simulink library "vehicleWeight_cl"  (R2022a)
settings: Solver=VariableStepAuto  StartTime=0.0  StopTime=10.0  RelTol=1e-3
undefined symbols (not defined in the file): env, VEHICLE, vhcl
libraries: vrlib x2, eulAng2RotMat_ul x1, eulDot x1, tethersMoment_cl x1, thrAttachPtKinematics_ul x1
settings Model: Creator=mcobb  LastModifiedBy=lhill8
settings SolverCC: AlgebraicLoopSolver=TrustRegion
settings DebuggingCC: UnconnectedInputMsg=warning  UnconnectedOutputMsg=warning  UnconnectedLineMsg=warning  SFMachineParentedDataDiag=warning  ArithmeticOperatorsInVariantConditions=warning
settings SFSimCC: CustomCodeUndefinedFunction=UseInterfaceOnly

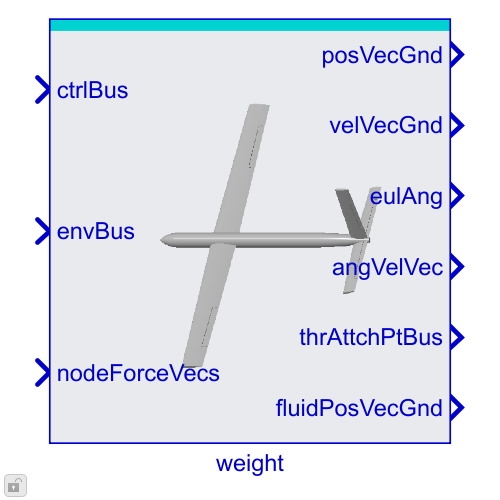
[thumbnail: Simulink's stored preview of the top-level diagram]
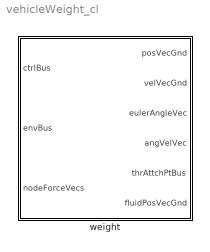
== system vehicleWeight_cl ==
  weight : Subsystem  VariantControl=strcmpi(VEHICLE,'vehicleManta2Rot')  mask{vcl=vhcl, rho=env.water.density.Value, grav=env.gravAccel.Value}
      mask prompts: vcl "Vehicle"; rho "Density"; grav "Gravity"
      mask DialogControl Container9 Prompt: General
      mask DialogControl Container5 Prompt: Vehicle object (OCT.vehicle)
      mask DialogControl ParameterGroupVar Prompt: Environment Object (OCT.env)
      mask Display:
      | image('kite2.PNG',[0 0 700 700]/4,'on')
      | 
      | port_label('input',1,'ctrlBus')
      | port_label('input',2,'envBus')
      | port_label('input',3,'nodeForceVecs')
      | 
      | port_label('output',1,'posVecGnd')
      | port_label('output',2,'velVecGnd')
      | port_label('output',3,'eulAng')
      | port_label('output',4,'angVelVec')
      | port_label('output',5,'thrAttchPtBus')
      | port_label('output',6,'fluidPosVecGnd')

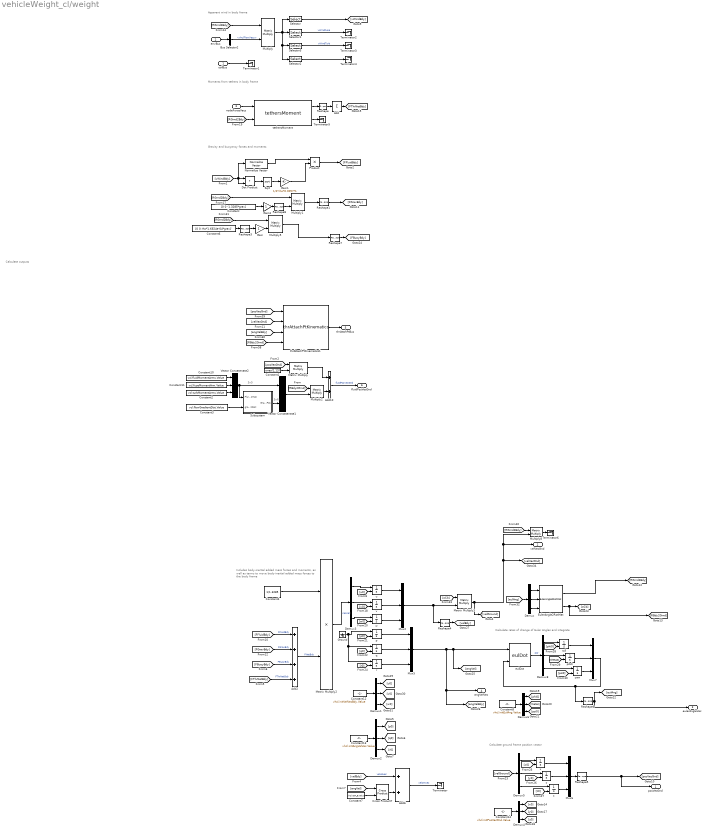
== system vehicleWeight_cl/weight ==
  note: 3x6
  note: 3x5
  note: Calculate outputs
  note: Apparent wind in body frame
  note: Gravity and buoyancy forces and moments
  note: Moments from tethers in body frame
  note: Calculate rates of change of Euler Angles and integrate
  note: Includes body-inertial added mass forces and moments,
      | as well as terms to move body-inertial added mass
      | forces to the body frame
  note: Calculate ground frame position vector
  ctrlBus : Inport
  envBus : Inport  Port=2  OutDataTypeStr=Bus: envBus
  nodeForceVecs : Inport  Port=3
  Add : Sum  Inputs=+  CollapseMode=Specified dimension  CollapseDim=2
  Add10 : Sum
  Add2 : Sum  Inputs=++++
  Add6 : Sum
  Bus Selector2 : BusSelector  OutputSignals=vhclFlowVecs
  Constant : Constant  Value=[0 0 -1.3285*grav]
  Constant1 : Constant  Value=ones(1,13)  VectorParams1D=off
  Constant10 : Constant  Value=vcl.fluidMomentArms.Value
  Constant11 : Constant  Value=vcl.fuseMomentArm.Value
  Constant12 : Constant  Value=vhcl.initVelVecBdy.Value
  Constant13 : Constant  Value=vhcl.initAngVelVec.Value
  Constant14 : Constant  Value=vhcl.initPosVecGnd.Value
  Constant2 : Constant  Value=vcl.turbMomentArms.Value
  Constant3 : Constant  Value=vcl.flowGradientDist.Value
  Constant4 : Constant  Value=1/1.3285  VectorParams1D=off
  Constant6 : Constant  Value=[0 0 rho*1.6924e-04*grav]'
  Constant7 : Constant  Value=vhcl.rCM_B.Value
  Constant8 : Constant  Value=vhcl.initEulAng.Value
  Cross Product7 : vrlib/Utilities/Cross Product
  Demux{,1..6,8} (8 alike) : Demux  Outputs=3
  Dot Product : DotProduct  OutDataTypeStr=Inherit: Inherit via internal rule
  EulerAngle2RotMat : eulAng2RotMat_ul/EulerAngle2RotMat  SystemSampleTime=-1  VariantActivationTime=update diagram  Latency=0  AutoFrameSizeCalculation=off
  Gain : Gain
  Gain1 : Gain  Gain=1/2*rho*0.0057*1
  Gain3 : Gain
  Ground : Ground
  Matrix Multiply : Product  Multiplication=Matrix(*)
  Matrix Multiply2 : Product
  Matrix Multiply3 : Product  Multiplication=Matrix(*)
  Multiply{,1..2,5,8} (5 alike) : Product  Multiplication=Matrix(*)
  Mux{2,5..7} (4 alike) : Mux  Inputs=3
  Normalize Vector : vrlib/Utilities/Normalize Vector  maxzero=0
  Product : Product
  Reshape : Reshape  OutputDimensionality=Customize  OutputDimensions=[3 vcl.numTethers.Value]
  Reshape{1,3..8} (7 alike) : Reshape  OutputDimensionality=Column vector (2-D)
  Selector : Selector  NumberOfDimensions=2  InputPortWidth=3  IndexOptions=Select all,Index vector (dialog)  Indices=[1 3],1  OutputSizes=1,1
  Selector1 : Selector  NumberOfDimensions=2  InputPortWidth=3  IndexOptions=Select all,Index vector (dialog)  Indices=[1 3],5  OutputSizes=1,1
  Selector2 : Selector  NumberOfDimensions=2  InputPortWidth=3  IndexOptions=Select all,Index vector (dialog)  Indices=[1 3],8:13  OutputSizes=1,1
  Selector3 : Selector  NumberOfDimensions=2  InputPortWidth=3  IndexOptions=Select all,Index vector (dialog)  Indices=[1 3],6:7  OutputSizes=1,1
  Sqrt : Sqrt
  Subsystem : Subsystem
  Terminator{,1..6} (7 alike) : Terminator
  Vector Concatenate1 : Concatenate  Mode=Multidimensional array  ConcatenateDimension=2
  Vector Concatenate2 : Concatenate  NumInputs=3  Mode=Multidimensional array  ConcatenateDimension=2
  eulDot : eulDot/eulDot  SystemSampleTime=-1  VariantActivationTime=update diagram  Latency=0  AutoFrameSizeCalculation=off
  p : Integrator  InitialConditionSource=external
  pitch : Integrator  InitialConditionSource=external
  q : Integrator  InitialConditionSource=external
  r : Integrator  InitialConditionSource=external
  roll : Integrator  InitialConditionSource=external
  tethersMoment : tethersMoment_cl/tethersMoment  arms=vcl.struct('OCT.thrAttch')
  thrAttachPtKinematics1 : thrAttachPtKinematics_ul/thrAttachPtKinematics  atchPts=vcl.struct('OCT.thrAttch')
  u : Integrator  InitialConditionSource=external
  v : Integrator  InitialConditionSource=external
  w : Integrator  InitialConditionSource=external
  x : Integrator  InitialConditionSource=external
  y : Integrator  InitialConditionSource=external
  yaw : Integrator  InitialConditionSource=external
  z : Integrator  InitialConditionSource=external
  posVecGnd : Outport  VectorParamsAs1DForOutWhenUnconnected=off
  velVecGnd : Outport  Port=2  VectorParamsAs1DForOutWhenUnconnected=off
  eulerAngleVec : Outport  Port=3  VectorParamsAs1DForOutWhenUnconnected=off
  angVelVec : Outport  Port=4  VectorParamsAs1DForOutWhenUnconnected=off
  thrAttchPtBus : Outport  Port=5  VectorParamsAs1DForOutWhenUnconnected=off
  fluidPosVecGnd : Outport  Port=6  VectorParamsAs1DForOutWhenUnconnected=off
  wires:
  thrAttachPtKinematics1/1 -> thrAttchPtBus/1
  Constant6/1 -> Reshape3/1
  Reshape3/1 -> Gain/1
  [RGrnd2Bdy] -> Multiply5/1
  Gain/1 -> Multiply5/2
  Multiply5/1 -> Reshape7/1
  Reshape7/1 -> [FBuoyBdy]
  Reshape1/1 -> [FGravBdy]
  Multiply1/1 -> Reshape1/1
  Constant/1 -> Gain3/1
  [RGrnd2Bdy] -> Multiply1/1
  Reshape8/1 -> Multiply1/2
  [RGrnd2Bdy] -> tethersMoment/2
  nodeForceVecs/1 -> tethersMoment/1
  tethersMoment/1 -> Reshape/1
  tethersMoment/2 -> Terminator5/1
  Reshape/1 -> Add/1
  Add/1 -> [FThrNetBdy]
  [RGrnd2Bdy] -> Multiply/1
  envBus/1 -> Bus Selector2/1
  Bus Selector2/1 -> Multiply/2  "<vhclFlowVecs>"
  Multiply/1 -> Selector/1, Selector2/1, Selector3/1, Selector1/1
  Selector/1 -> [vWindBdy]
  Selector1/1 -> Terminator2/1  "vWindFuse"
  Selector2/1 -> Terminator4/1
  [posVecGnd] -> thrAttachPtKinematics1/1
  [velVecGnd] -> thrAttachPtKinematics1/2
  [angVelBdy] -> thrAttachPtKinematics1/3
  [RBdy2Grnd] -> thrAttachPtKinematics1/4
  Constant10/1 -> Vector Concatenate2/1
  Constant11/1 -> Vector Concatenate2/2
  Vector Concatenate2/1 -> Vector Concatenate1/1, Subsystem/1(FluidCentPosMat)
  Constant3/1 -> Subsystem/2(gradientDist)
  Subsystem/1(GradientFlowPos) -> Vector Concatenate1/2
  Vector Concatenate1/1 -> Multiply2/2
  [RBdy2Grnd] -> Multiply2/1
  Multiply2/1 -> Add10/2
  Matrix Multiply/1 -> Add10/1
  Add10/1 -> fluidPosVecGnd/1  "fluidPosVecGnd"
  Constant1/1 -> Matrix Multiply/2
  [posVecGnd] -> Matrix Multiply/1
  Constant2/1 -> Vector Concatenate2/3
  Selector3/1 -> Terminator3/1  "vWindTurb"
  Gain3/1 -> Reshape8/1
  [vWindBdy] -> Normalize Vector/1, Dot Product/2, Dot Product/1
  Dot Product/1 -> Sqrt/1
  Normalize Vector/1 -> Product/1
  Sqrt/1 -> Gain1/1
  Product/1 -> [FFluidBdy]
  Reshape4/1 -> [velBdy]
  [r0] -> r/2
  [angVel] -> Cross Product7/1
  q/1 -> Mux5/2
  Demux6/1 -> [phi0]
  [q0] -> q/2
  Demux2/3 -> [r0]
  roll/1 -> Mux7/1
  [p0] -> p/2
  r/1 -> Mux5/3
  y/1 -> Mux6/2
  Demux5/1 -> x/1
  w/1 -> Mux2/3
  v/1 -> Mux2/2
  u/1 -> Mux2/1
  Demux3/2 -> v/1
  Constant12/1 -> Demux1/1
  Ground/1 -> r/1, q/1, p/1
  Demux3/3 -> w/1
  Demux/2 -> EulerAngle2RotMat/2
  z/1 -> Mux6/3
  Constant14/1 -> Demux4/1
  Demux1/2 -> [v0]
  Demux3/1 -> u/1
  Constant7/1 -> Cross Product7/2
  Demux1/3 -> [w0]
  Demux2/2 -> [q0]
  Demux1/1 -> [u0]
  Demux/1 -> EulerAngle2RotMat/1
  Constant4/1 -> Matrix Multiply2/1
  x/1 -> Mux6/1
  Mux7/1 -> eulDot/2, Reshape6/1
  [theta0] -> pitch/2
  Demux/3 -> EulerAngle2RotMat/3
  Matrix Multiply2/1 -> Demux3/1  "caccel"
  Mux2/1 -> Matrix Multiply3/2, Reshape4/1
  [velBdy] -> Add6/1  "velLEvec"
  Demux8/2 -> pitch/1
  Cross Product7/1 -> Add6/2
  Demux2/1 -> [p0]
  Demux6/2 -> [theta0]
  [oCb] -> Matrix Multiply3/1
  [u0] -> u/2
  Demux4/3 -> [z0]
  Demux4/1 -> [x0]
  [phi0] -> roll/2
  Demux5/3 -> z/1
  Add6/1 -> Terminator/1  "velCMvec"
  [x0] -> x/2
  p/1 -> Mux5/1
  [y0] -> y/2
  [z0] -> z/2
  [eulAng] -> Demux/1
  Constant8/1 -> Demux6/1
  [w0] -> w/2
  Demux4/2 -> [y0]
  [velGround] -> Demux5/1
  Demux6/3 -> [psi0]
  [psi0] -> yaw/2
  Constant13/1 -> Demux2/1
  pitch/1 -> Mux7/2
  Demux8/3 -> yaw/1
  Demux8/1 -> roll/1
  Mux6/1 -> Reshape5/1
  [v0] -> v/2
  eulDot/1 -> Demux8/1  "pqr"
  Demux5/2 -> y/1
  yaw/1 -> Mux7/3
  [FThrNetBdy] -> Add2/4  "FThrNetBdy"
  [FGravBdy] -> Add2/2  "FGravBdy"
  Add2/1 -> Matrix Multiply2/2  "FNetBdy"
  [FFluidBdy] -> Add2/1  "FFluidBdy"
  [FBuoyBdy] -> Add2/3  "FBuoyBdy"
  Reshape5/1 -> posVecGnd/1, [posVecGnd]
  Multiply8/1 -> Terminator6/1
  [RGrnd2Bdy] -> Multiply8/1
  Matrix Multiply3/1 -> Multiply8/2, velVecGnd/1, [velVecGnd], [velGround]
  Reshape6/1 -> eulerAngleVec/1, [eulAng]
  Mux5/1 -> [angVelBdy], angVelVec/1, eulDot/1, [angVel]
  EulerAngle2RotMat/1 -> [RGrnd2Bdy]
  EulerAngle2RotMat/2 -> [RBdy2Grnd], [oCb]
  ctrlBus/1 -> Terminator1/1
  Gain1/1 -> Product/2

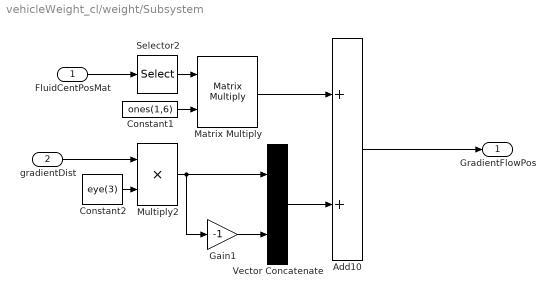
== system vehicleWeight_cl/weight/Subsystem ==
  FluidCentPosMat : Inport
  gradientDist : Inport  Port=2
  Add10 : Sum
  Constant1 : Constant  Value=ones(1,6)  VectorParams1D=off
  Constant2 : Constant  Value=eye(3)
  Gain1 : Gain  Gain=-1
  Matrix Multiply : Product  Multiplication=Matrix(*)
  Multiply2 : Product
  Selector2 : Selector  NumberOfDimensions=2  InputPortWidth=3  IndexOptions=Select all,Index vector (dialog)  Indices=[1 3],5  OutputSizes=1,1
  Vector Concatenate : Concatenate  Mode=Multidimensional array  ConcatenateDimension=2
  GradientFlowPos : Outport  VectorParamsAs1DForOutWhenUnconnected=off
  wires:
  FluidCentPosMat/1 -> Selector2/1
  Vector Concatenate/1 -> Add10/2
  Selector2/1 -> Matrix Multiply/1
  Multiply2/1 -> Gain1/1, Vector Concatenate/1
  Constant1/1 -> Matrix Multiply/2
  Matrix Multiply/1 -> Add10/1
  Gain1/1 -> Vector Concatenate/2
  Constant2/1 -> Multiply2/2
  Add10/1 -> GradientFlowPos/1
  gradientDist/1 -> Multiply2/1
